simulink model "11_pmsmMBD_V1"  (R2019b)
settings: Solver=ode45  StartTime=0.0  StopTime=1  RelTol=1e-3
undefined symbols (not defined in the file or in its folder): DiscIntNeverNeededParam
libraries: powerlib x4, simulink x1
settings Model: Creator=liuzhong  LastModifiedBy=李瑾年
settings SFSimCC: CustomCodeUndefinedFunction=UseInterfaceOnly

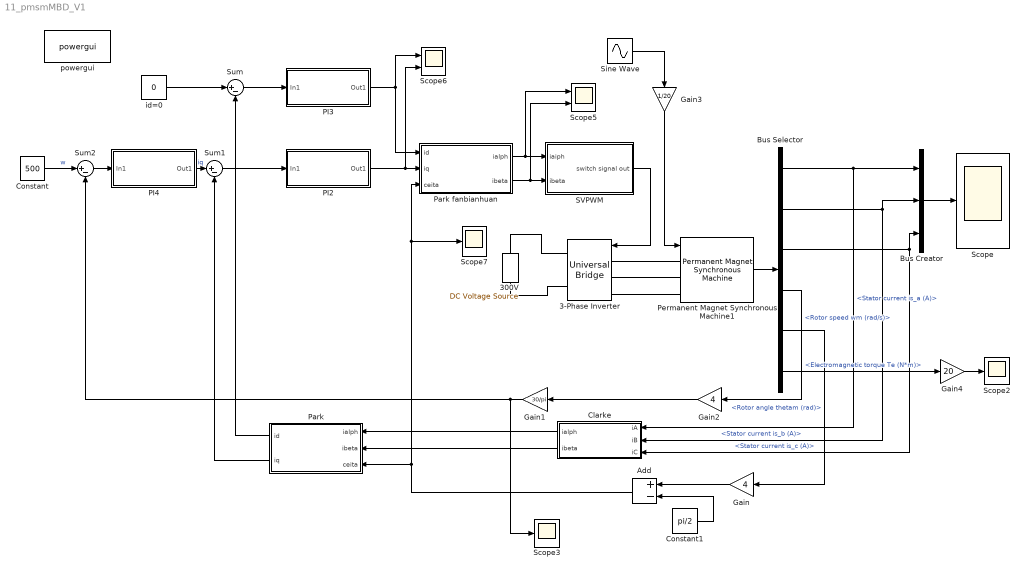
== system 11_pmsmMBD_V1 ==
  3-Phase Inverter : powerlib/Power Electronics/Universal Bridge  Arms=3  SnubberResistance=1e5  SnubberCapacitance=inf  Device=IGBT / Diodes  Ron=1e-3  Lon=0  ForwardVoltages="[  0  0  ]"  ForwardVoltage=0  GTOparameters=[ 10e-6 , 20e-6 ]  IGBTparameters=[ 1e-6 , 2e-6 ]  Measurements=None  Measurements_2=None  converterType=Rectifier
      settings: SourceProductName=Simscape Electrical
  300V : powerlib/Electrical Sources/DC Voltage Source  Amplitude=300  Measurements=Voltage
      settings: SourceProductName=Simscape Electrical
  Add : Sum  Inputs=+-
  Bus Creator : BusCreator  Inputs=3
  Bus Selector : BusSelector  OutputSignals=Stator current is_a (A),Stator current is_b (A),Stator current is_c (A),Rotor speed wm (rad/s),Rotor angle thetam (rad),Electromagnetic torque Te (N*m)
  Clarke : Subsystem
  Constant : Constant  Value=500
  Constant1 : Constant  Value=pi/2
  Gain : Gain  Gain=4
  Gain1 : Gain  Gain=30/pi
  Gain2 : Gain  Gain=4
  Gain3 : Gain  Gain=1/20
  Gain4 : Gain  Gain=20
  PI2 : Subsystem
  PI3 : Subsystem
  PI4 : Subsystem
  Park : Subsystem
  Park fanbianhuan : Subsystem
  Permanent Magnet Synchronous Machine1 : powerlib/Machines/Permanent Magnet Synchronous Machine  NbPhases=3  FluxDistribution=Sinusoidal  RotorType=Round  MechanicalLoad=Torque Tm  PresetModel=No  ShowDetailedParameters=on  MeasurementBus=off  Resistance=0.901  Inductance=8.5e-3  dqInductances=[0.02682 0.02682]  La=0.006365  MachineConstant=Torque Constant (N.m / A_peak)  Flux=0.13333  VoltageCst=96.736  TorqueCst=0.8  Flat=120  Mechanical=[0.00012 0.0008 4]  PolePairs=2  InitialConditions=[0,0, 0,0]  InitialConditions5ph=[0 0 0 0 0 0]  RefAngle=90 degrees behind phase A axis (modified Park)  IterativeDiscreteModel=Trapezoidal non iterative  TsBlock=-1  TsPowergui=0
  SVPWM : Subsystem
  Scope{,2..3,7} (4 alike) : Scope
  Scope5 : Scope  NumInputPorts=2
  Scope6 : Scope  NumInputPorts=2
  Sine Wave : Sin  Amplitude=2  Frequency=pi/2  SampleTime=0
  Sum : Sum  Inputs=|+-
  Sum1 : Sum  Inputs=|+-
  Sum2 : Sum  Inputs=|+-
  id=0 : Constant  Value=0
  powergui : powerlib/powergui  Priority=1  SimulationMode=Discrete  SampleTime=1e-6  frequency=60  Iterations=50  frequencyindice=0  Pbase=100e6  ErrMax=1e-4  UnitsV=kV  UnitsW=MW  buscounter=0  FunctionMessages=off  echomessages=off  EnableUseOfTLC=off  CurrentSourceSwitches=off  DisableSnubberDevices=off  DisableRonSwitches=off  DisableVfSwitches=off  DisplayEquations=off  AutomaticDiscreteSolvers=off  SolverType=Tustin/Backward Euler (TBE)  Interpol=off  ExternalGateDelay=off  methode=off  Ts=100  x0status=blocks  SPID=on  SwTol=0  HookPort=off  NonlinearTolerance=0  nMaxIteration=15  ContinueOnMaxIteration=off  RestoreLinks=warning  ResistiveCurrentMeasurement=off  Frange=[0:2:500]  Ylog=off  Xlog=on  ShowGrid=off  save=off  variable=ZData  structure=0  ZoomFFT=off  StartTime=0.0  cycles=1  DisplayStyle=1  fundamental=60  FreqAxis=off  MaxFrequency=1000  frequencyindicesteady=1  RmsSteady=1  display=off
      settings: SourceProductName=Simscape Electrical
  wires:
  Clarke/1(ialph) -> Park/1(ialph)
  Clarke/2(ibeta) -> Park/2(ibeta)
  id=0/1 -> Sum/1
  Sum1/1 -> PI2/1(In1)
  Park fanbianhuan/1(ialph) -> SVPWM/1(iaiph), Scope5/1
  Park fanbianhuan/2("ibeta ") -> SVPWM/2(ibeta), Scope5/2
  Sine Wave/1 -> Gain3/1
  SVPWM/1(switch signal out) -> 3-Phase Inverter/1
  Permanent Magnet Synchronous Machine1/1 -> Bus Selector/1
  Bus Selector/1 -> Bus Creator/1, Clarke/1(iA)  "<Stator current is_a (A)>"
  Bus Selector/2 -> Bus Creator/2, Clarke/2(iB)  "<Stator current is_b (A)>"
  Bus Selector/3 -> Bus Creator/3, Clarke/3(iC)  "<Stator current is_c (A)>"
  PI3/1(Out1) -> Scope6/1, Park fanbianhuan/1(id)
  PI2/1(Out1) -> Scope6/2, Park fanbianhuan/2(iq)
  Sum/1 -> PI3/1(In1)
  Bus Selector/4 -> Gain2/1  "<Rotor speed wm (rad/s)>"
  Bus Creator/1 -> Scope/1
  Bus Selector/6 -> Gain4/1  "<Electromagnetic torque Te (N*m)>"
  Sum2/1 -> PI4/1(In1)
  Bus Selector/5 -> Gain/1  "<Rotor angle thetam (rad)>"
  PI4/1(Out1) -> Sum1/1  "iq"
  Constant/1 -> Sum2/1  "w"
  Park/2(iq) -> Sum1/2
  Park/1(id) -> Sum/2
  Add/1 -> Scope7/1, Park fanbianhuan/3(ceita), Park/3(ceita)
  Gain1/1 -> Sum2/2, Scope3/1
  Gain2/1 -> Gain1/1
  Gain/1 -> Add/1
  Constant1/1 -> Add/2
  Gain3/1 -> Permanent Magnet Synchronous Machine1/1
  Gain4/1 -> Scope2/1
  connections:
  Permanent Magnet Synchronous Machine1/LConn1 -- 3-Phase Inverter/LConn1
  Permanent Magnet Synchronous Machine1/LConn2 -- 3-Phase Inverter/LConn2
  Permanent Magnet Synchronous Machine1/LConn3 -- 3-Phase Inverter/LConn3
  300V/RConn1 -- 3-Phase Inverter/RConn1
  3-Phase Inverter/RConn2 -- 300V/LConn1

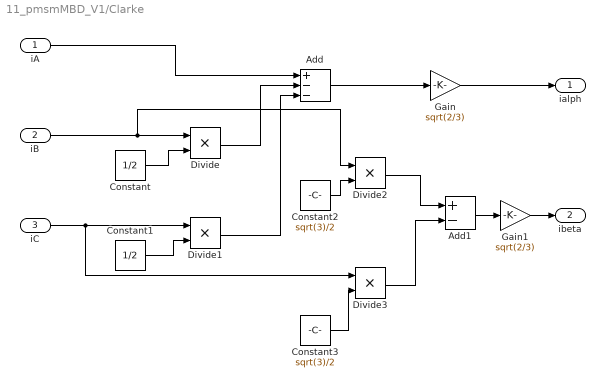
== system 11_pmsmMBD_V1/Clarke ==
  iA : Inport
  iB : Inport  Port=2
  iC : Inport  Port=3
  Add : Sum  Inputs=+--
  Add1 : Sum  Inputs=+-
  Constant : Constant  Value=1/2
  Constant1 : Constant  Value=1/2
  Constant2 : Constant  Value=sqrt(3)/2
  Constant3 : Constant  Value=sqrt(3)/2
  Divide{,1..3} (4 alike) : Product  Inputs=**
  Gain : Gain  Gain=sqrt(2/3)
  Gain1 : Gain  Gain=sqrt(2/3)
  ialph : Outport  VectorParamsAs1DForOutWhenUnconnected=off
  ibeta : Outport  Port=2  VectorParamsAs1DForOutWhenUnconnected=off
  wires:
  Add/1 -> Gain/1
  iA/1 -> Add/1
  iB/1 -> Divide/1, Divide2/1
  Constant/1 -> Divide/2
  Divide/1 -> Add/2
  iC/1 -> Divide1/1, Divide3/1
  Constant1/1 -> Divide1/2
  Divide1/1 -> Add/3
  Constant2/1 -> Divide2/2
  Divide2/1 -> Add1/1
  Constant3/1 -> Divide3/2
  Divide3/1 -> Add1/2
  Add1/1 -> Gain1/1
  Gain/1 -> ialph/1
  Gain1/1 -> ibeta/1

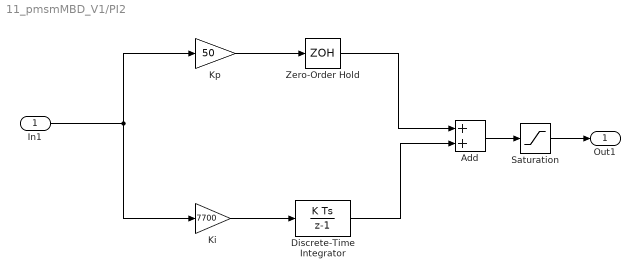
== system 11_pmsmMBD_V1/PI2 ==
  In1 : Inport
  Add : Sum
  Discrete-Time Integrator : DiscreteIntegrator  SampleTime=50e-6  LimitOutput=on  UpperSaturationLimit=500  LowerSaturationLimit=-500  ICPrevOutput=DiscIntNeverNeededParam  ICPrevScaledInput=DiscIntNeverNeededParam
  Ki : Gain  Gain=7700
  Kp : Gain  Gain=50
  Saturation : Saturate  UpperLimit=300  LowerLimit=-300
  Zero-Order Hold : ZeroOrderHold  SampleTime=50e-6
  Out1 : Outport  VectorParamsAs1DForOutWhenUnconnected=off
  wires:
  Kp/1 -> Zero-Order Hold/1
  Ki/1 -> Discrete-Time Integrator/1
  In1/1 -> Ki/1, Kp/1
  Zero-Order Hold/1 -> Add/1
  Discrete-Time Integrator/1 -> Add/2
  Add/1 -> Saturation/1
  Saturation/1 -> Out1/1

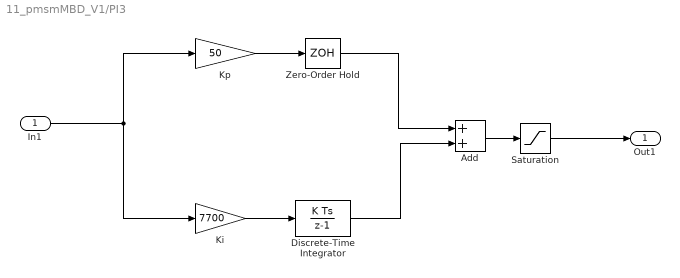
== system 11_pmsmMBD_V1/PI3 ==
  In1 : Inport
  Add : Sum
  Discrete-Time Integrator : DiscreteIntegrator  SampleTime=50e-6  LimitOutput=on  UpperSaturationLimit=500  LowerSaturationLimit=-500  ICPrevOutput=DiscIntNeverNeededParam  ICPrevScaledInput=DiscIntNeverNeededParam
  Ki : Gain  Gain=7700
  Kp : Gain  Gain=50
  Saturation : Saturate  UpperLimit=300  LowerLimit=-300
  Zero-Order Hold : ZeroOrderHold  SampleTime=50e-6
  Out1 : Outport  VectorParamsAs1DForOutWhenUnconnected=off
  wires:
  Kp/1 -> Zero-Order Hold/1
  Ki/1 -> Discrete-Time Integrator/1
  In1/1 -> Ki/1, Kp/1
  Zero-Order Hold/1 -> Add/1
  Discrete-Time Integrator/1 -> Add/2
  Add/1 -> Saturation/1
  Saturation/1 -> Out1/1

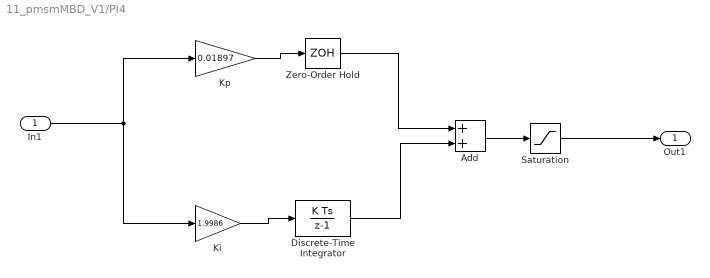
== system 11_pmsmMBD_V1/PI4 ==
  In1 : Inport
  Add : Sum
  Discrete-Time Integrator : DiscreteIntegrator  SampleTime=50e-6  LimitOutput=on  UpperSaturationLimit=300  LowerSaturationLimit=-300  ICPrevOutput=DiscIntNeverNeededParam  ICPrevScaledInput=DiscIntNeverNeededParam
  Ki : Gain  Gain=1.9986
  Kp : Gain  Gain=0.01897
  Saturation : Saturate  UpperLimit=300  LowerLimit=-300
  Zero-Order Hold : ZeroOrderHold  SampleTime=50e-6
  Out1 : Outport  VectorParamsAs1DForOutWhenUnconnected=off
  wires:
  Kp/1 -> Zero-Order Hold/1
  Ki/1 -> Discrete-Time Integrator/1
  In1/1 -> Ki/1, Kp/1
  Zero-Order Hold/1 -> Add/1
  Discrete-Time Integrator/1 -> Add/2
  Add/1 -> Saturation/1
  Saturation/1 -> Out1/1

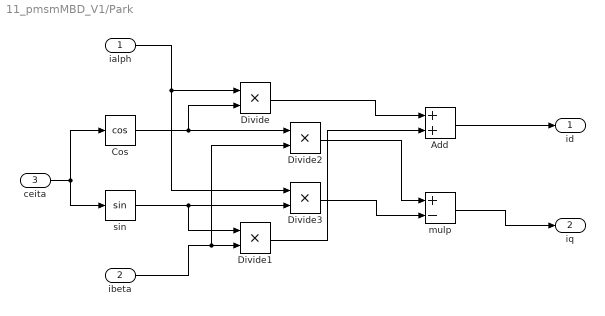
== system 11_pmsmMBD_V1/Park ==
  ialph : Inport
  ibeta : Inport  Port=2
  ceita : Inport  Port=3
  Add : Sum
  Cos : Trigonometry  Operator=cos
  Divide{,1..3} (4 alike) : Product  Inputs=**
  mulp : Sum  Inputs=+-
  sin : Trigonometry
  id : Outport  VectorParamsAs1DForOutWhenUnconnected=off
  iq : Outport  Port=2  VectorParamsAs1DForOutWhenUnconnected=off
  wires:
  ceita/1 -> sin/1, Cos/1
  ialph/1 -> Divide/1, Divide3/1
  Cos/1 -> Divide2/1, Divide/2
  sin/1 -> Divide1/1, Divide3/2
  ibeta/1 -> Divide2/2, Divide1/2
  Divide/1 -> Add/1
  Divide1/1 -> Add/2
  Add/1 -> id/1
  Divide2/1 -> mulp/1
  Divide3/1 -> mulp/2
  mulp/1 -> iq/1

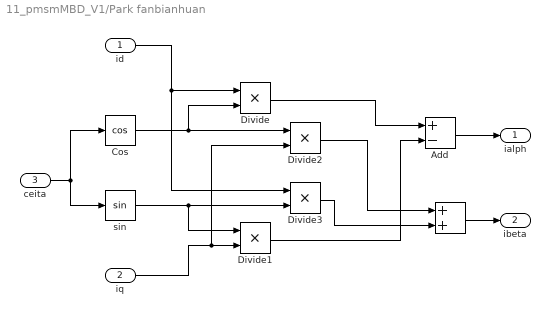
== system 11_pmsmMBD_V1/Park fanbianhuan ==
  id : Inport
  iq : Inport  Port=2
  ceita : Inport  Port=3
  " " : Sum
  Add : Sum  Inputs=+-
  Cos : Trigonometry  Operator=cos
  Divide{,1..3} (4 alike) : Product  Inputs=**
  sin : Trigonometry
  ialph : Outport  VectorParamsAs1DForOutWhenUnconnected=off
  "ibeta " : Outport  Port=2  VectorParamsAs1DForOutWhenUnconnected=off
  wires:
  ceita/1 -> sin/1, Cos/1
  id/1 -> Divide/1, Divide3/1
  Cos/1 -> Divide2/1, Divide/2
  sin/1 -> Divide1/1, Divide3/2
  iq/1 -> Divide2/2, Divide1/2
  Divide/1 -> Add/1
  Divide1/1 -> Add/2
  Add/1 -> ialph/1
  Divide2/1 -> " "/1
  Divide3/1 -> " "/2
  " "/1 -> "ibeta "/1

== system 11_pmsmMBD_V1/SVPWM ==
  iaiph : Inport
  ibeta : Inport  Port=2
  compute time : Subsystem
  "select location " : Subsystem
  switch signal : Subsystem
  switch signal out : Outport  VectorParamsAs1DForOutWhenUnconnected=off
  wires:
  iaiph/1 -> compute time/2(Ualph), "select location "/1(Uaiph)
  ibeta/1 -> "select location "/2(Ubeta), compute time/3(Ubeta)
  "select location "/1(location) -> compute time/1(location), switch signal/1(location)
  compute time/1(t1) -> switch signal/2(T1)
  compute time/2(t2) -> switch signal/3(T2)
  compute time/3(t0) -> switch signal/4(T0)
  switch signal/1(signal) -> switch signal out/1

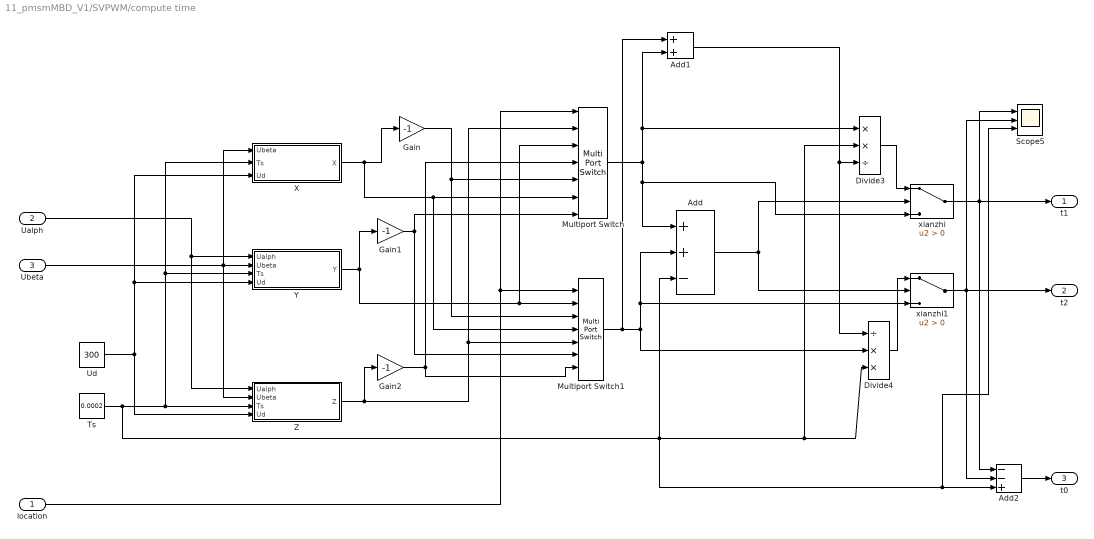
== system 11_pmsmMBD_V1/SVPWM/compute time ==
  location : Inport
  Ualph : Inport  Port=2
  Ubeta : Inport  Port=3
  Add : Sum  Inputs=++-
  Add1 : Sum
  Add2 : Sum  Inputs=--+
  Divide3 : Product  Inputs=**/
  Divide4 : Product  Inputs=/**
  Gain : Gain  Gain=-1
  Gain1 : Gain  Gain=-1
  Gain2 : Gain  Gain=-1
  Multiport Switch : MultiPortSwitch  Inputs=6  DiagnosticForDefault=None
  Multiport Switch1 : MultiPortSwitch  Inputs=6  DiagnosticForDefault=None
  Scope5 : Scope  NumInputPorts=3
  Ts : Constant  Value=0.0002
  Ud : Constant  Value=300
  X : Subsystem
  Y : Subsystem
  Z : Subsystem
  xianzhi : Switch  Criteria=u2 > Threshold
  xianzhi1 : Switch  Criteria=u2 > Threshold
  t1 : Outport  VectorParamsAs1DForOutWhenUnconnected=off
  t2 : Outport  Port=2  VectorParamsAs1DForOutWhenUnconnected=off
  t0 : Outport  Port=3  VectorParamsAs1DForOutWhenUnconnected=off
  wires:
  Ualph/1 -> Y/1(Ualph), Z/1(Ualph)
  Ubeta/1 -> X/1(Ubeta), Y/2(Ubeta), Z/2(Ubeta)
  Ts/1 -> Add/3, Divide3/2, Divide4/3, Scope5/3, Add2/3, X/2(Ts), Y/3(Ts), Z/3(Ts)
  Ud/1 -> Z/4(Ud), X/3(Ud), Y/4(Ud)
  Y/1(Y) -> Gain1/1, Multiport Switch/3, Multiport Switch1/2
  Z/1(Z) -> Gain2/1, Multiport Switch1/5, Multiport Switch/2
  Gain/1 -> Multiport Switch1/3, Multiport Switch/5
  Gain2/1 -> Multiport Switch1/7, Multiport Switch/4
  X/1(X) -> Gain/1, Multiport Switch1/4, Multiport Switch/6
  Gain1/1 -> Multiport Switch/7, Multiport Switch1/6
  Add/1 -> xianzhi1/2, xianzhi/2
  Multiport Switch/1 -> Divide3/1, Add1/2, xianzhi/3, Add/1
  Multiport Switch1/1 -> Add1/1, Divide4/2, Add/2, xianzhi1/3
  xianzhi/1 -> Scope5/1, Add2/1, t1/1
  xianzhi1/1 -> Scope5/2, Add2/2, t2/1
  Add1/1 -> Divide3/3, Divide4/1
  Divide3/1 -> xianzhi/1
  Divide4/1 -> xianzhi1/1
  location/1 -> Multiport Switch/1, Multiport Switch1/1
  Add2/1 -> t0/1

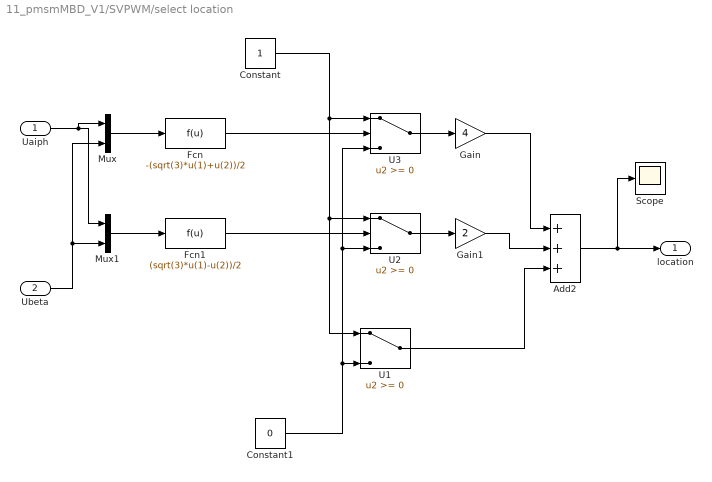
== system 11_pmsmMBD_V1/SVPWM/select location  ==
  Uaiph : Inport
  Ubeta : Inport  Port=2
  Add2 : Sum  Inputs=+++
  Constant : Constant
  Constant1 : Constant  Value=0
  Fcn : Fcn  Expr=-(sqrt(3)*u(1)+u(2))/2
  Fcn1 : Fcn  Expr=(sqrt(3)*u(1)-u(2))/2
  Gain : Gain  Gain=4
  Gain1 : Gain  Gain=2
  Mux : Mux  Inputs=2
  Mux1 : Mux  Inputs=2
  Scope : Scope
  U1 : Switch
  U2 : Switch
  U3 : Switch
  location : Outport  VectorParamsAs1DForOutWhenUnconnected=off
  wires:
  Constant1/1 -> U1/3, U2/3, U3/3
  Constant/1 -> U3/1, U2/1, U1/1
  Fcn/1 -> U3/2
  Fcn1/1 -> U2/2
  U2/1 -> Gain1/1
  U1/1 -> Add2/3
  Gain/1 -> Add2/1
  Gain1/1 -> Add2/2
  Add2/1 -> Scope/1, location/1
  U3/1 -> Gain/1
  Uaiph/1 -> Mux1/1, Mux/1
  Mux/1 -> Fcn/1
  Ubeta/1 -> Mux1/2, Mux/2
  Mux1/1 -> Fcn1/1

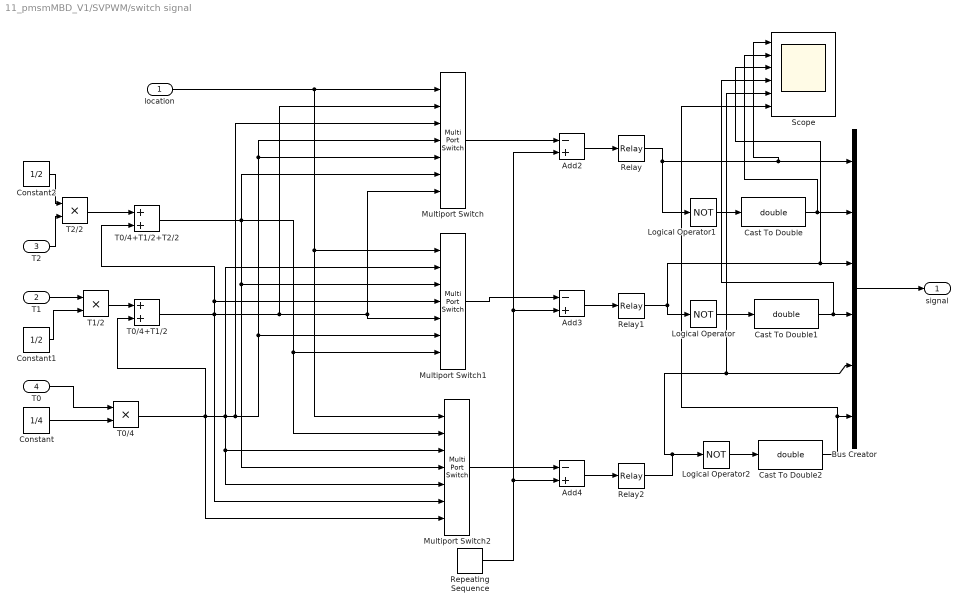
== system 11_pmsmMBD_V1/SVPWM/switch signal ==
  location : Inport
  T1 : Inport  Port=2
  T2 : Inport  Port=3
  T0 : Inport  Port=4
  Add2 : Sum  Inputs=-+
  Add3 : Sum  Inputs=-+
  Add4 : Sum  Inputs=-+
  Bus Creator : BusCreator  Inputs=6
  Cast To Double : DataTypeConversion  OutDataTypeStr=double
  Cast To Double1 : DataTypeConversion  OutDataTypeStr=double
  Cast To Double2 : DataTypeConversion  OutDataTypeStr=double
  Constant : Constant  Value=1/4
  Constant1 : Constant  Value=1/2
  Constant2 : Constant  Value=1/2
  Logical Operator : Logic  Operator=NOT  AllPortsSameDT=off  OutDataTypeStr=boolean
  Logical Operator1 : Logic  Operator=NOT  AllPortsSameDT=off  OutDataTypeStr=boolean
  Logical Operator2 : Logic  Operator=NOT  AllPortsSameDT=off  OutDataTypeStr=boolean
  Multiport Switch : MultiPortSwitch  Inputs=6  DiagnosticForDefault=None
  Multiport Switch1 : MultiPortSwitch  Inputs=6  DiagnosticForDefault=None
  Multiport Switch2 : MultiPortSwitch  Inputs=6  DiagnosticForDefault=None
  Relay : Relay
  Relay1 : Relay
  Relay2 : Relay
  Repeating Sequence : simulink/Sources/Repeating Sequence  rep_seq_t=[0 0.0001 0.0002]  rep_seq_y=[0 0.0001 0]
  Scope : Scope  NumInputPorts=6
  T0/4 : Product  Inputs=**
  T0/4+T1/2 : Sum
  T0/4+T1/2+T2/2 : Sum
  T1/2 : Product  Inputs=**
  T2/2 : Product  Inputs=**
  signal : Outport  VectorParamsAs1DForOutWhenUnconnected=off
  wires:
  location/1 -> Multiport Switch/1, Multiport Switch1/1, Multiport Switch2/1
  Constant/1 -> T0/4/2
  T0/1 -> T0/4/1
  T0/4/1 -> Multiport Switch2/5, Multiport Switch2/3, Multiport Switch/3, Multiport Switch/4, Multiport Switch/5, Multiport Switch1/6, Multiport Switch1/2, Multiport Switch2/7, T0/4+T1/2/2
  T2/1 -> T2/2/2
  T0/4+T1/2/1 -> Multiport Switch1/5, Multiport Switch/7, Multiport Switch/2, T0/4+T1/2+T2/2/2, Multiport Switch1/4, Multiport Switch2/6
  Multiport Switch/1 -> Add2/1
  Multiport Switch1/1 -> Add3/1
  Multiport Switch2/1 -> Add4/1
  T1/2/1 -> T0/4+T1/2/1
  T1/1 -> T1/2/1
  Constant1/1 -> T1/2/2
  Constant2/1 -> T2/2/1
  T2/2/1 -> T0/4+T1/2+T2/2/1
  Repeating Sequence/1 -> Add3/2, Add2/2, Add4/2
  Add2/1 -> Relay/1
  Add4/1 -> Relay2/1
  Add3/1 -> Relay1/1
  Relay1/1 -> Logical Operator/1, Scope/3, Bus Creator/3
  Relay/1 -> Logical Operator1/1, Scope/1, Bus Creator/1
  Logical Operator1/1 -> Cast To Double/1
  Relay2/1 -> Bus Creator/5, Scope/5, Logical Operator2/1
  Bus Creator/1 -> signal/1
  Logical Operator/1 -> Cast To Double1/1
  Cast To Double/1 -> Scope/2, Bus Creator/2
  Cast To Double1/1 -> Scope/4, Bus Creator/4
  Cast To Double2/1 -> Scope/6, Bus Creator/6
  Logical Operator2/1 -> Cast To Double2/1
  T0/4+T1/2+T2/2/1 -> Multiport Switch1/3, Multiport Switch2/4, Multiport Switch/6, Multiport Switch1/7, Multiport Switch2/2

== system 11_pmsmMBD_V1/SVPWM/compute time/X ==
  Ubeta : Inport
  Ts : Inport  Port=2
  Ud : Inport  Port=3
  Constant1 : Constant  Value=sqrt(3)
  Divide : Product  Inputs=**
  Divide1 : Product  Inputs=**/
  X : Outport  VectorParamsAs1DForOutWhenUnconnected=off
  wires:
  Ubeta/1 -> Divide/1
  Constant1/1 -> Divide/2
  Divide/1 -> Divide1/1
  Ts/1 -> Divide1/2
  Ud/1 -> Divide1/3
  Divide1/1 -> X/1

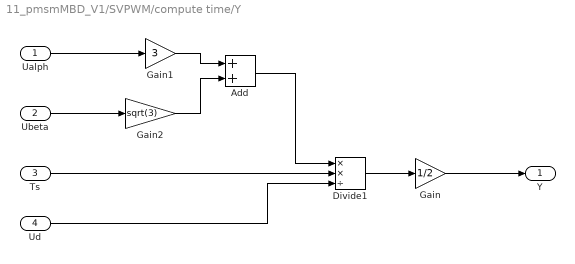
== system 11_pmsmMBD_V1/SVPWM/compute time/Y ==
  Ualph : Inport
  Ubeta : Inport  Port=2
  Ts : Inport  Port=3
  Ud : Inport  Port=4
  Add : Sum
  Divide1 : Product  Inputs=**/
  Gain : Gain  Gain=1/2
  Gain1 : Gain  Gain=3
  Gain2 : Gain  Gain=sqrt(3)
  Y : Outport  VectorParamsAs1DForOutWhenUnconnected=off
  wires:
  Ud/1 -> Divide1/3
  Ts/1 -> Divide1/2
  Divide1/1 -> Gain/1
  Ubeta/1 -> Gain2/1
  Ualph/1 -> Gain1/1
  Gain1/1 -> Add/1
  Gain2/1 -> Add/2
  Add/1 -> Divide1/1
  Gain/1 -> Y/1

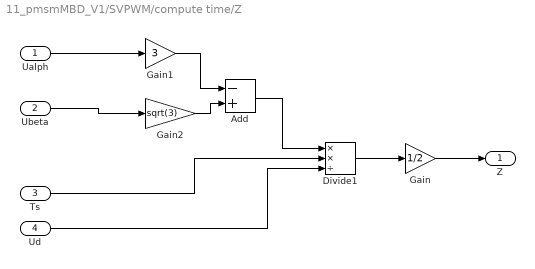
== system 11_pmsmMBD_V1/SVPWM/compute time/Z ==
  Ualph : Inport
  Ubeta : Inport  Port=2
  Ts : Inport  Port=3
  Ud : Inport  Port=4
  Add : Sum  Inputs=-+
  Divide1 : Product  Inputs=**/
  Gain : Gain  Gain=1/2
  Gain1 : Gain  Gain=3
  Gain2 : Gain  Gain=sqrt(3)
  Z : Outport  VectorParamsAs1DForOutWhenUnconnected=off
  wires:
  Gain2/1 -> Add/2
  Add/1 -> Divide1/1
  Ualph/1 -> Gain1/1
  Ud/1 -> Divide1/3
  Gain/1 -> Z/1
  Divide1/1 -> Gain/1
  Ts/1 -> Divide1/2
  Gain1/1 -> Add/1
  Ubeta/1 -> Gain2/1
